simulink model "SRAM"  (R2017b)
settings: Solver=FixedStepAuto  StartTime=0.0  StopTime=1  FixedStep=0.02  RelTol=1e-3  EnableMultiTasking=on
undefined symbols (not defined in the file or in its folder): tfinal
settings Model: Creator=niestma  LastModifiedBy=Soutrik
settings DataIOCC: LimitDataPoints=on
settings OptimizationCC: LifeSpan=inf
settings DebuggingCC: AllowSymbolicDim=off  SFUnexpectedBacktrackingDiag=warning  SFNoUnconditionalDefaultTransitionDiag=warning  SFExecutionAtInitializationDiag=none
settings ModelReferenceCC: PropagateSignalLabelsOutOfModel=off
settings CodeAppCC: StateflowObjectComments=on
settings GRTTargetCC: TargetLangStandard=C89/C90 (ANSI)
settings ConfigComp: CovMetricSettings=dw  CovHtmlReporting=on  CovSaveCumulativeToWorkspaceVar=on  CovSaveSingleToWorkspaceVar=on  CovExternalEMLEnable=off

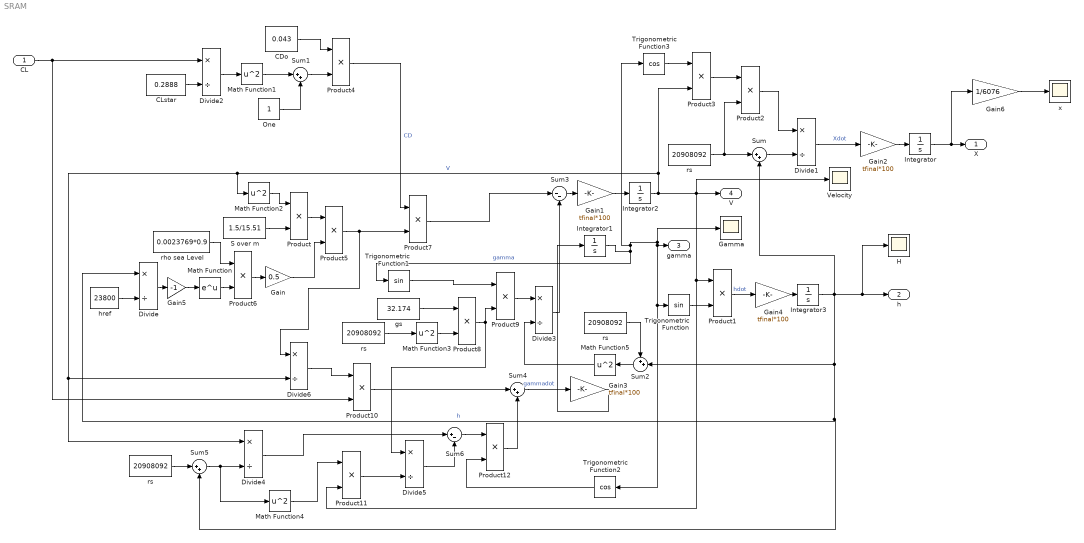
== system SRAM ==
  CL : Inport
  CDo : Constant  Value=0.043
  CLstar : Constant  Value=0.2888
  Divide{,1..6} (7 alike) : Product  Inputs=*/
  Gain : Gain  Gain=0.5
  Gain{1..4} (4 alike) : Gain  Gain=tfinal*100
  Gain5 : Gain  Gain=-1
  Gain6 : Gain  Gain=1/6076
  Gamma : Scope
  H : Scope
  Integrator : Integrator
  Integrator1 : Integrator
  Integrator2 : Integrator  InitialCondition=11000
  Integrator3 : Integrator  InitialCondition=100000
  Math Function : Math  SaturateOnIntegerOverflow=on
  Math Function{1..5} (5 alike) : Math  Operator=square  SaturateOnIntegerOverflow=on
  One : Constant
  Product{,1..12} (13 alike) : Product
  S over m : Constant  Value=1.5/15.51
  Sum{,1,4..5} (4 alike) : Sum  Inputs=|++
  Sum2 : Sum  Inputs=++|
  Sum3 : Sum  Inputs=|--
  Sum6 : Sum  Inputs=|+-
  Trigonometric Function : Trigonometry
  Trigonometric Function1 : Trigonometry
  Trigonometric Function2 : Trigonometry  Operator=cos
  Trigonometric Function3 : Trigonometry  Operator=cos
  Velocity : Scope
  gs : Constant  Value=32.174
  href : Constant  Value=23800
  rho sea Level : Constant  Value=0.0023769*0.9
  rs : Constant  Value=20908092
  "rs " : Constant  Value=20908092
  "rs  " : Constant  Value=20908092
  "rs   " : Constant  Value=20908092
  x : Scope
  X : Outport
  h : Outport  Port=2
  gamma : Outport  Port=3
  V : Outport  Port=4
  wires:
  Trigonometric Function/1 -> Product1/2
  Product1/1 -> Gain4/1  "hdot"
  Integrator1/1 -> gamma/1, Trigonometric Function2/1, Trigonometric Function/1, Gamma/1, Trigonometric Function3/1, Trigonometric Function1/1  "gamma"
  Integrator2/1 -> Divide6/2, Divide4/1, Math Function2/1, Product3/2, Velocity/1, V/1, Product11/2, Product1/1  "V"
  Integrator3/1 -> H/1, h/1, Sum/2, Sum2/2, Sum5/2, Divide/1  "h"
  rs/1 -> Product2/2, Sum/1
  Sum/1 -> Divide1/2
  Divide1/1 -> Gain2/1  "Xdot"
  Product2/1 -> Divide1/1
  Product3/1 -> Product2/1
  Trigonometric Function3/1 -> Product3/1
  CL/1 -> Product10/2, Divide2/1
  CLstar/1 -> Divide2/2
  Divide2/1 -> Math Function1/1
  Math Function1/1 -> Sum1/1
  One/1 -> Sum1/2
  Sum1/1 -> Product4/2
  CDo/1 -> Product4/1
  S over m/1 -> Product/2
  Math Function2/1 -> Product/1
  Product/1 -> Product5/1
  href/1 -> Divide/2
  Math Function/1 -> Product6/2
  rho sea Level/1 -> Product6/1
  Product6/1 -> Gain/1
  Gain/1 -> Product5/2
  Product5/1 -> Divide6/1, Product7/2
  Product4/1 -> Product7/1  "CD"
  "rs "/1 -> Math Function3/1
  Math Function3/1 -> Product8/2
  gs/1 -> Product8/1
  Product8/1 -> Divide5/1, Product9/2
  Trigonometric Function1/1 -> Product9/1
  Product9/1 -> Divide3/1
  Sum2/1 -> Math Function5/1
  "rs  "/1 -> Sum2/1
  Sum3/1 -> Gain1/1
  Divide3/1 -> Sum3/2
  Product7/1 -> Sum3/1
  Sum4/1 -> Gain3/1  "gammadot"
  Product10/1 -> Sum4/1
  "rs   "/1 -> Sum5/1
  Sum5/1 -> Math Function4/1, Divide4/2
  Math Function4/1 -> Product11/1
  Product11/1 -> Divide5/2
  Divide4/1 -> Sum6/1
  Divide5/1 -> Sum6/2
  Sum6/1 -> Product12/1
  Product12/1 -> Sum4/2
  Trigonometric Function2/1 -> Product12/2
  Integrator/1 -> Gain6/1, X/1
  Gain2/1 -> Integrator/1
  Gain1/1 -> Integrator2/1
  Gain3/1 -> Integrator1/1
  Gain4/1 -> Integrator3/1
  Math Function5/1 -> Divide3/2
  Gain5/1 -> Math Function/1
  Divide/1 -> Gain5/1
  Gain6/1 -> x/1
  Divide6/1 -> Product10/1
